simulink model "hdlcoder_singlePh_spwm"  (R2022b)
settings: Solver=VariableStepAuto  StartTime=0.0  StopTime=0.05  RelTol=1e-3
libraries: simulink x1, hdlsllib x1, dspsrcs4 x1
settings Model: Creator=BAYINDIR  LastModifiedBy=BAYINDIR
settings OptimizationCC: BlockReduction=off  ConditionallyExecuteInputs=off

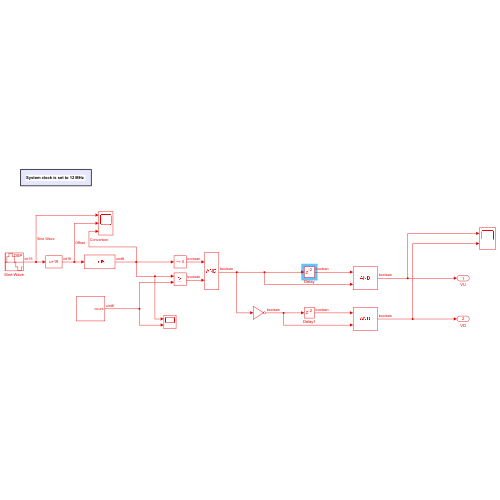
[thumbnail: Simulink's stored preview of the top-level diagram]
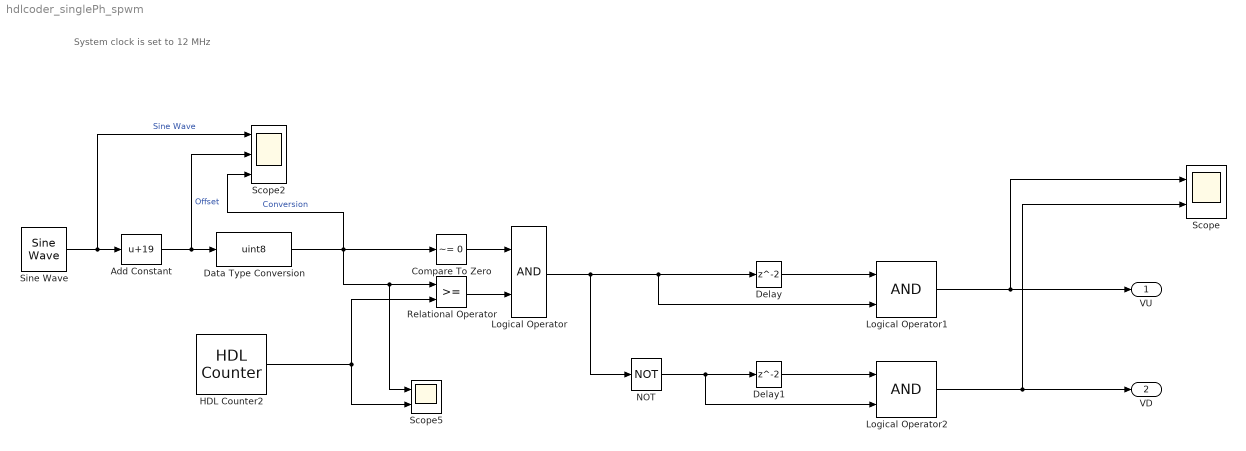
== system hdlcoder_singlePh_spwm ==
  note: System clock is set to 12 MHz
  Add Constant : Bias  Bias=19  SaturateOnIntegerOverflow=off
  Compare To Zero : simulink/Logic and Bit Operations/Compare To Zero  relop=~=  OutDataTypeStr=boolean
  Data Type Conversion : DataTypeConversion  OutMin=[0]  OutMax=[120]  OutDataTypeStr=uint8  SaturateOnIntegerOverflow=off  RndMeth=Floor
  Delay : Delay  InitialCondition=0  UseCircularBuffer=on
  Delay1 : Delay  InitialCondition=0  UseCircularBuffer=on
  HDL Counter2 : hdlsllib/Sources/HDL Counter  CountType=Count limited  CountInit=0  CountStep=1  CountMax=48  CountFromType=Initial value  CountFrom=0  CountResetPort=off  CountLoadPort=off  CountEnbPort=off  CountDirPort=off  CountHitOutputPort=off  CountDataType=Unsigned  CountWordLen=8  CountFracLen=0  CountSampTime=1/12e6
  Logical Operator : Logic  AllPortsSameDT=off  OutDataTypeStr=boolean
  Logical Operator1 : Logic  AllPortsSameDT=off  OutDataTypeStr=boolean
  Logical Operator2 : Logic  AllPortsSameDT=off  OutDataTypeStr=boolean
  NOT : Logic  Operator=NOT  IconShape=distinctive  AllPortsSameDT=off  OutDataTypeStr=boolean
  Relational Operator : RelationalOperator  OutDataTypeStr=boolean  RndMeth=Simplest  InputSameDT=off
  Scope : Scope  NumInputPorts=2
  Scope2 : Scope  NumInputPorts=3
  Scope5 : Scope  NumInputPorts=2
  Sine Wave : dspsrcs4/Sine Wave  Amplitude=19  Frequency=60  Phase=0  SampleMode=Discrete  OutComplex=Real  CompMethod=Table lookup  TableSize=Memory  SampleTime=1/12e6  SamplesPerFrame=1  ResetState=Restart at time zero  OutputFrames=off  dataType=Fixed-point  wordLen=16  udDataType=sfix(16)  fracBitsMode=User-defined  numFracBits=0  OutDataTypeStr=fixdt(1,16,0)  LastOutDataTypeStr=fixdt(1,16,0)
  VU : Outport  VectorParamsAs1DForOutWhenUnconnected=off
  VD : Outport  Port=2  VectorParamsAs1DForOutWhenUnconnected=off
  wires:
  Sine Wave/1 -> Add Constant/1, Scope2/1  "Sine Wave"
  Relational Operator/1 -> Logical Operator/2
  Compare To Zero/1 -> Logical Operator/1
  HDL Counter2/1 -> Scope5/2, Relational Operator/2
  Delay/1 -> Logical Operator1/1
  Add Constant/1 -> Scope2/2, Data Type Conversion/1  "Offset"
  Data Type Conversion/1 -> Scope5/1, Relational Operator/1, Compare To Zero/1, Scope2/3  "Conversion"
  Logical Operator2/1 -> VD/1, Scope/2
  NOT/1 -> Logical Operator2/2, Delay1/1
  Logical Operator/1 -> Logical Operator1/2, Delay/1, NOT/1
  Logical Operator1/1 -> Scope/1, VU/1
  Delay1/1 -> Logical Operator2/1
